simulink model "theta_correction"  (R2018a)
settings: Solver=VariableStepAuto  StartTime=0.0  StopTime=10.0  FixedStep=0.01  RelTol=1e-3
settings Model: Creator=blond  LastModifiedBy=blond

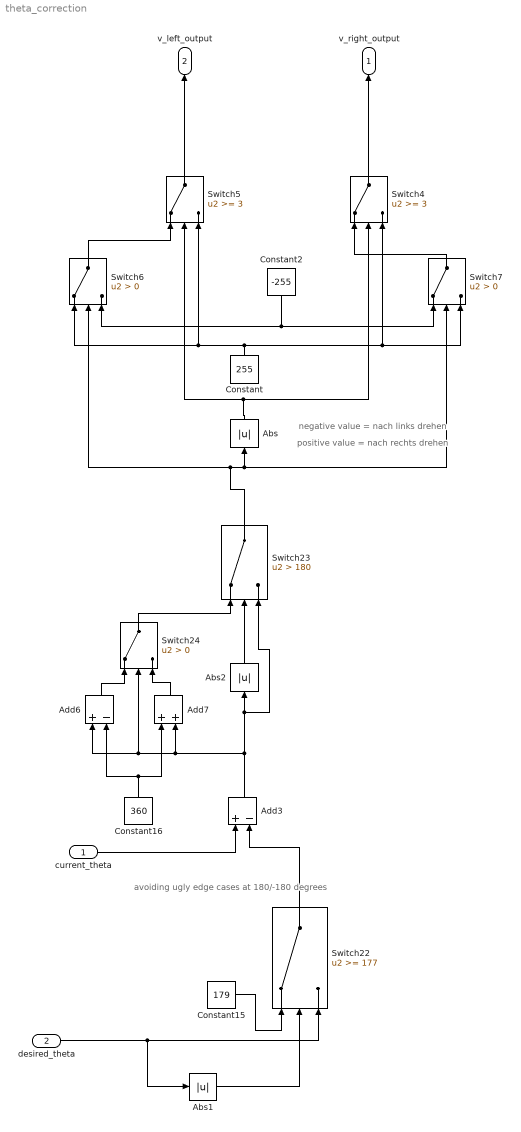
== system theta_correction ==
  note: positive value = nach rechts drehen
  note: negative value = nach links drehen
  note: avoiding ugly edge cases at
      | 180/-180 degrees
  current_theta : Inport
  desired_theta : Inport  Port=2
  Abs : Abs  ZeroCross=off
  Abs1 : Abs  ZeroCross=off
  Abs2 : Abs  ZeroCross=off
  Add3 : Sum  Inputs=+-
  Add6 : Sum  Inputs=+-
  Add7 : Sum
  Constant : Constant  Value=255
  Constant15 : Constant  Value=179
  Constant16 : Constant  Value=360
  Constant2 : Constant  Value=-255
  Switch22 : Switch  Threshold=177  ZeroCross=off
  Switch23 : Switch  Criteria=u2 > Threshold  Threshold=180  ZeroCross=off
  Switch24 : Switch  Criteria=u2 > Threshold  ZeroCross=off
  Switch4 : Switch  Threshold=3  ZeroCross=off
  Switch5 : Switch  Threshold=3  ZeroCross=off
  Switch6 : Switch  Criteria=u2 > Threshold  ZeroCross=off
  Switch7 : Switch  Criteria=u2 > Threshold  ZeroCross=off
  v_right_output : Outport
  v_left_output : Outport  Port=2
  wires:
  Add7/1 -> Switch24/3
  Abs1/1 -> Switch22/2
  Add6/1 -> Switch24/1
  Constant15/1 -> Switch22/1
  Switch6/1 -> Switch5/1
  Constant/1 -> Switch7/3, Switch4/3, Switch6/1, Switch5/3
  Add3/1 -> Add7/2, Add6/1, Switch24/2, Switch23/3, Abs2/1
  Constant16/1 -> Add6/2, Add7/1
  Abs2/1 -> Switch23/2
  Switch23/1 -> Abs/1, Switch7/2, Switch6/2
  Switch5/1 -> v_left_output/1
  Switch22/1 -> Add3/2
  Switch7/1 -> Switch4/1
  Switch24/1 -> Switch23/1
  Switch4/1 -> v_right_output/1
  Abs/1 -> Switch4/2, Switch5/2
  desired_theta/1 -> Switch22/3, Abs1/1
  current_theta/1 -> Add3/1
  Constant2/1 -> Switch7/1, Switch6/3
